simulink model "lab6_part3"  (R2022b)
settings: Solver=VariableStepAuto  StartTime=0.0  StopTime=20.0  RelTol=1e-3
settings Model: Creator=ADMIN  LastModifiedBy=ADMIN

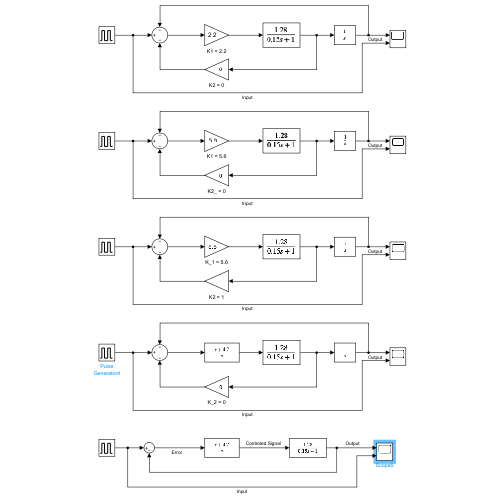
[thumbnail: Simulink's stored preview of the top-level diagram]
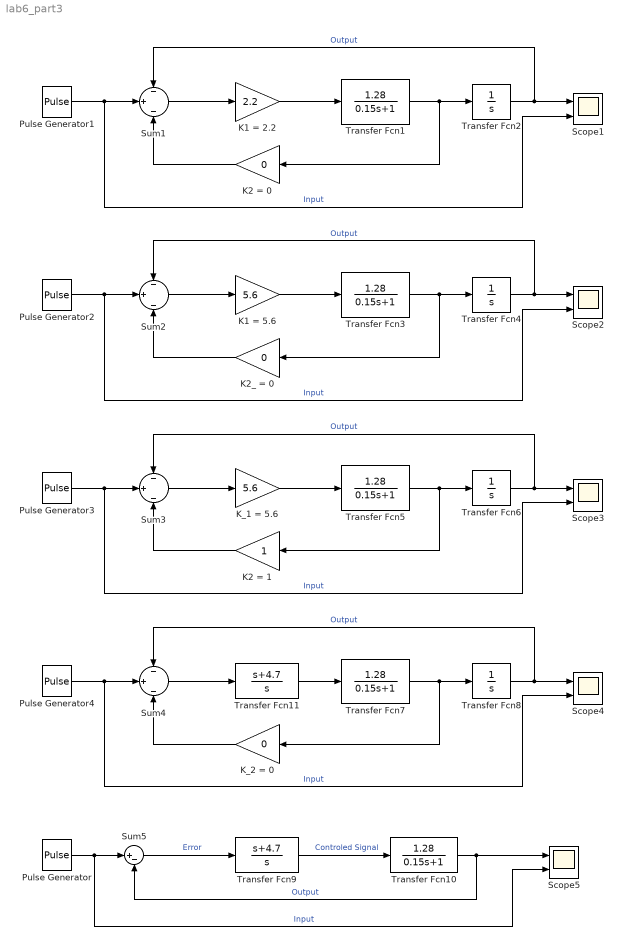
== system lab6_part3 ==
  K1 = 2.2 : Gain  Gain=2.2
  K1 = 5.6 : Gain  Gain=5.6
  K2 = 0 : Gain  Gain=0
  K2 = 1 : Gain
  K2_ = 0 : Gain  Gain=0
  K_1 = 5.6 : Gain  Gain=5.6
  K_2 = 0 : Gain  Gain=0
  Pulse Generator{,1..4} (5 alike) : DiscretePulseGenerator  PulseType=Time based  Amplitude=3  Period=10  PulseWidth=50
  Scope{1..5} (5 alike) : Scope  NumInputPorts=2
  Sum{1..4} (4 alike) : Sum  Inputs=-|+|-
  Sum5 : Sum  Inputs=|+-
  Transfer Fcn{1,3,5,7,10} (5 alike) : TransferFcn  Numerator=[1.28]  Denominator=[0.15 1]
  Transfer Fcn11 : TransferFcn  Numerator=[1 4.7]  Denominator=[1 0]
  Transfer Fcn{2,4,6,8} (4 alike) : TransferFcn  Denominator=[1 0]
  Transfer Fcn9 : TransferFcn  Numerator=[1 4.7]  Denominator=[1 0]
  wires:
  Transfer Fcn1/1 -> K2 = 0/1, Transfer Fcn2/1
  K2 = 0/1 -> Sum1/3
  K1 = 2.2/1 -> Transfer Fcn1/1
  Transfer Fcn2/1 -> Sum1/1, Scope1/1  "Output"
  Pulse Generator1/1 -> Scope1/2, Sum1/2  "Input"
  Sum1/1 -> K1 = 2.2/1
  Pulse Generator2/1 -> Scope2/2, Sum2/2  "Input"
  Sum2/1 -> K1 = 5.6/1
  Transfer Fcn4/1 -> Sum2/1, Scope2/1  "Output"
  Transfer Fcn3/1 -> K2_ = 0/1, Transfer Fcn4/1
  K1 = 5.6/1 -> Transfer Fcn3/1
  K2_ = 0/1 -> Sum2/3
  K_1 = 5.6/1 -> Transfer Fcn5/1
  K2 = 1/1 -> Sum3/3
  Sum3/1 -> K_1 = 5.6/1
  Transfer Fcn5/1 -> K2 = 1/1, Transfer Fcn6/1
  Pulse Generator3/1 -> Scope3/2, Sum3/2  "Input"
  Transfer Fcn6/1 -> Sum3/1, Scope3/1  "Output"
  Pulse Generator4/1 -> Scope4/2, Sum4/2  "Input"
  Sum4/1 -> Transfer Fcn11/1
  Transfer Fcn7/1 -> K_2 = 0/1, Transfer Fcn8/1
  K_2 = 0/1 -> Sum4/3
  Transfer Fcn11/1 -> Transfer Fcn7/1
  Transfer Fcn8/1 -> Sum4/1, Scope4/1  "Output"
  Transfer Fcn9/1 -> Transfer Fcn10/1  "Controled Signal"
  Transfer Fcn10/1 -> Sum5/2, Scope5/1  "Output"
  Sum5/1 -> Transfer Fcn9/1  "Error"
  Pulse Generator/1 -> Scope5/2, Sum5/1  "Input"
